simulink model "SimulationCSI"  (R2023b)
settings: Solver=ode1  StartTime=0.0  StopTime=10.0  FixedStep=out_rate  RelTol=1e-3
InitFcn:
  | init
values from neighbouring files (symbols this model uses):
  dtheta_0 = 0    [DK_init.m]    (also in LQR_init.m; init.m)
  dz_0 = 0    [DK_init.m]    (also in LQR_init.m; init.m)
  theta_0 = 0    [DK_init.m]    (also in LQR_init.m; init.m)
  z_0 = 200    [DK_init.m]    (also in LQR_init.m; init.m = 0)
settings Model: Creator=franc  LastModifiedBy=franc

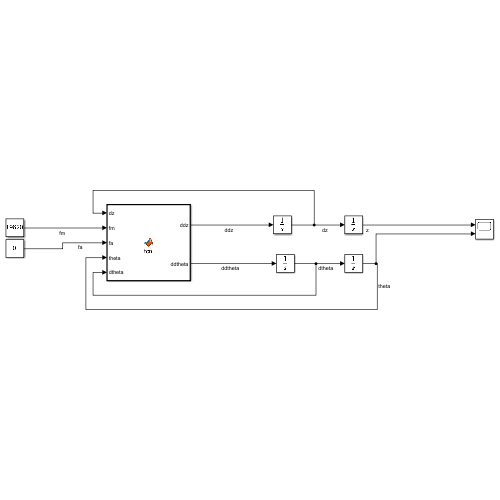
[thumbnail: Simulink's stored preview of the top-level diagram]
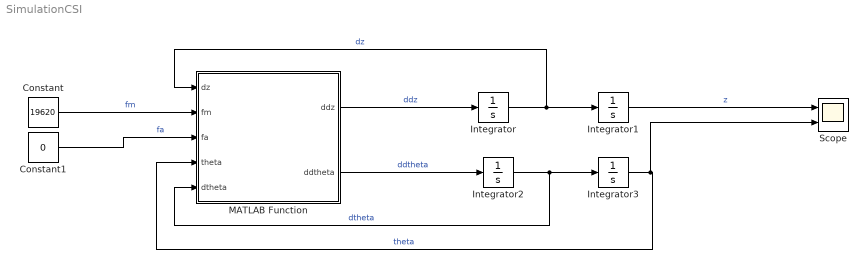
== system SimulationCSI ==
  Constant : Constant  Value=19620
  Constant1 : Constant  Value=0
  Integrator : Integrator  InitialCondition=dz_0
  Integrator1 : Integrator  InitialCondition=z_0
  Integrator2 : Integrator  InitialCondition=dtheta_0
  Integrator3 : Integrator  InitialCondition=theta_0
  MATLAB Function : MATLAB Function  TreatAsAtomicUnit=on
  Scope : Scope  NumInputPorts=2
  wires:
  MATLAB Function/1(ddz) -> Integrator/1  "ddz"
  Integrator/1 -> MATLAB Function/1(dz), Integrator1/1  "dz"
  MATLAB Function/2(ddtheta) -> Integrator2/1  "ddtheta"
  Integrator2/1 -> MATLAB Function/5(dtheta), Integrator3/1  "dtheta"
  Integrator3/1 -> Scope/2, MATLAB Function/4(theta)  "theta"
  Constant/1 -> MATLAB Function/2(fm)  "fm"
  Constant1/1 -> MATLAB Function/3(fa)  "fa"
  Integrator1/1 -> Scope/1  "z"

== matlab function SimulationCSI/MATLAB Function ==
  data: dz input; fm input; fa input; ddz output; ddtheta output; theta input; dtheta input; s_param parameter
function [ddz, ddtheta] = fcn(dz, fm, fa, theta, dtheta, s_param)
%% Rename params
J = s_param.J;     
m = s_param.m;     
b = s_param.b;      
beta = s_param.beta;    
g = s_param.g;     
l = s_param.l;   

%% Dynamic equations
ddz = -b/m * dz + fm/m * cos(theta) -g;
ddtheta = -beta/J * dtheta + 2 * l/J * fa;
end
